simulink library "Electric_Heater"  (Simulink 7.6)
settings: Solver=ode45  StartTime=0.0  StopTime=10.0  RelTol=1e-3
libraries: carnot x1
settings Model: Creator=lena.frank  LastModifiedBy=drhf

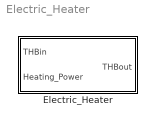
== system Electric_Heater ==
  Electric_Heater : Subsystem
      mask Type: Electric Heater
      mask Description: Heats the mass flow defined by the thermo-hydraulic bus with an electric power [W] entering the block.
      mask Help: web(fullfile(path_carnot('help'),'electric_heating.html'),'-helpbrowser')
      mask Display:
      | plot(0,0,100,100,[50,50,60,40,50],[55,40,70,60,90],[59,50],[48,40])
      | port_label('input',1,'THB')
      | port_label('input',2,'Qdot')
      | port_label('output',1,'THB')

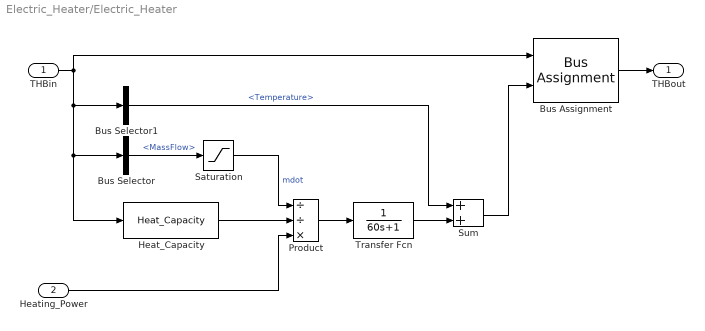
== system Electric_Heater/Electric_Heater ==
  THBin : Inport
  Heating_Power : Inport  Port=2
  Bus Assignment : BusAssignment  AssignedSignals=Temperature
  Bus Selector : BusSelector  OutputSignals=MassFlow
  Bus Selector1 : BusSelector  OutputSignals=Temperature
  Heat_Capacity : carnot/Basic/Material_Properties/Heat_Capacity  SystemSampleTime=-1  VariantObject=CarlibClassic  INPUTARGUMENTS=THB  DEBUGLEVEL=DEBUGLEVEL  MAXTOTALWARNINGS=inf  MAXCONSECUTIVEWARNINGS=inf  WRITETOFILE=0  FILENAME='errors.txt'
  Product : Product  Inputs=//*  SaturateOnIntegerOverflow=on  InputSameDT=on  OutDataTypeStr=Inherit: Same as first input
  Saturation : Saturate  UpperLimit=inf  LowerLimit=1e-5
  Sum : Sum  SaturateOnIntegerOverflow=on  InputSameDT=on  OutDataTypeStr=Inherit: Same as first input
  Transfer Fcn : TransferFcn  Denominator=[60 1]
  THBout : Outport  InitialOutput=0
  wires:
  THBin/1 -> Bus Assignment/1, Heat_Capacity/1, Bus Selector/1, Bus Selector1/1
  Product/1 -> Transfer Fcn/1
  Saturation/1 -> Product/1  "mdot"
  Heat_Capacity/1 -> Product/2
  Heating_Power/1 -> Product/3
  Transfer Fcn/1 -> Sum/2
  Bus Assignment/1 -> THBout/1
  Bus Selector/1 -> Saturation/1  "<MassFlow>"
  Bus Selector1/1 -> Sum/1  "<Temperature>"
  Sum/1 -> Bus Assignment/2
